simulink model "ITL_Basico"  (R2015a)
settings: Solver=ode45  StartTime=0.0  StopTime=10.0  RelTol=1e-3
settings Model: Creator=user  LastModifiedBy=user

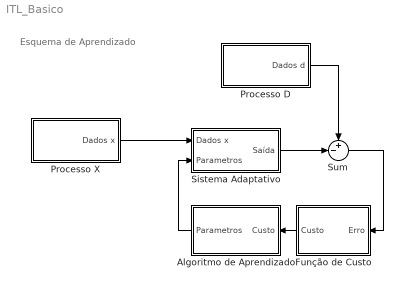
== system ITL_Basico ==
  note: Esquema de Aprendizado
  Algoritmo de Aprendizado : Subsystem
  Função de Custo : Subsystem
  Processo D : Subsystem
  Processo X : Subsystem
  Sistema Adaptativo : Subsystem
  Sum : Sum  Inputs=+-|
  wires:
  Sistema Adaptativo/1(Saída) -> Sum/2
  Sum/1 -> Função de Custo/1(Erro)
  Função de Custo/1(Custo) -> Algoritmo de Aprendizado/1(Custo)
  Algoritmo de Aprendizado/1(Parametros) -> Sistema Adaptativo/2(Parametros)
  Processo X/1(Dados x) -> Sistema Adaptativo/1(Dados x)
  Processo D/1(Dados d) -> Sum/1

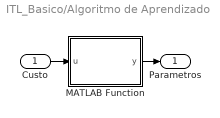
== system ITL_Basico/Algoritmo de Aprendizado ==
  Custo : Inport
  MATLAB Function : MATLAB Function  TreatAsAtomicUnit=on
  Parametros : Outport
  wires:
  Custo/1 -> MATLAB Function/1(u)
  MATLAB Function/1(y) -> Parametros/1

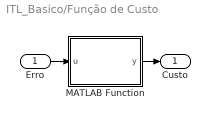
== system ITL_Basico/Função de Custo ==
  Erro : Inport
  MATLAB Function : MATLAB Function  TreatAsAtomicUnit=on
  Custo : Outport
  wires:
  Erro/1 -> MATLAB Function/1(u)
  MATLAB Function/1(y) -> Custo/1

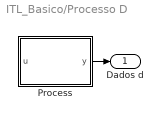
== system ITL_Basico/Processo D ==
  Process : MATLAB Function  TreatAsAtomicUnit=on
  Dados d : Outport
  wires:
  Process/1(y) -> Dados d/1

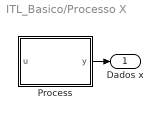
== system ITL_Basico/Processo X ==
  Process : MATLAB Function  TreatAsAtomicUnit=on
  Dados x : Outport
  wires:
  Process/1(y) -> Dados x/1

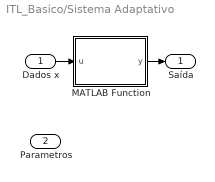
== system ITL_Basico/Sistema Adaptativo ==
  Dados x : Inport
  Parametros : Inport  Port=2
  MATLAB Function : MATLAB Function  TreatAsAtomicUnit=on
  Saída : Outport
  wires:
  Dados x/1 -> MATLAB Function/1(u)
  MATLAB Function/1(y) -> Saída/1

== matlab function ITL_Basico/Função de Custo/MATLAB Function ==
  data: u input; y output
function y = fcn(u)
%#codegen

y = u;

== matlab function ITL_Basico/Sistema Adaptativo/MATLAB Function ==
  data: u input; y output
function y = fcn(u)
%#codegen

y = u;

== matlab function ITL_Basico/Algoritmo de Aprendizado/MATLAB Function ==
  data: u input; y output
function y = fcn(u)
%#codegen

y = u;

== matlab function ITL_Basico/Processo X/Process ==
  data: u input; y output
function y = fcn(u)
%#codegen

y = u;

== matlab function ITL_Basico/Processo D/Process ==
  data: u input; y output
function y = fcn(u)
%#codegen

y = u;
